simulink model "AngualarVelcoityToRepTests"  (Simulink 8.3)
settings: Solver=ode3  StartTime=0.0  StopTime=9.0  FixedStep=0.01  RelTol=1e-3
settings Model: Creator=user  LastModifiedBy=philip
settings OptimizationCC: ExpressionDepthLimit=2147483647
settings DebuggingCC: FcnCallInpInsideContextMsg=UseLocalSettings

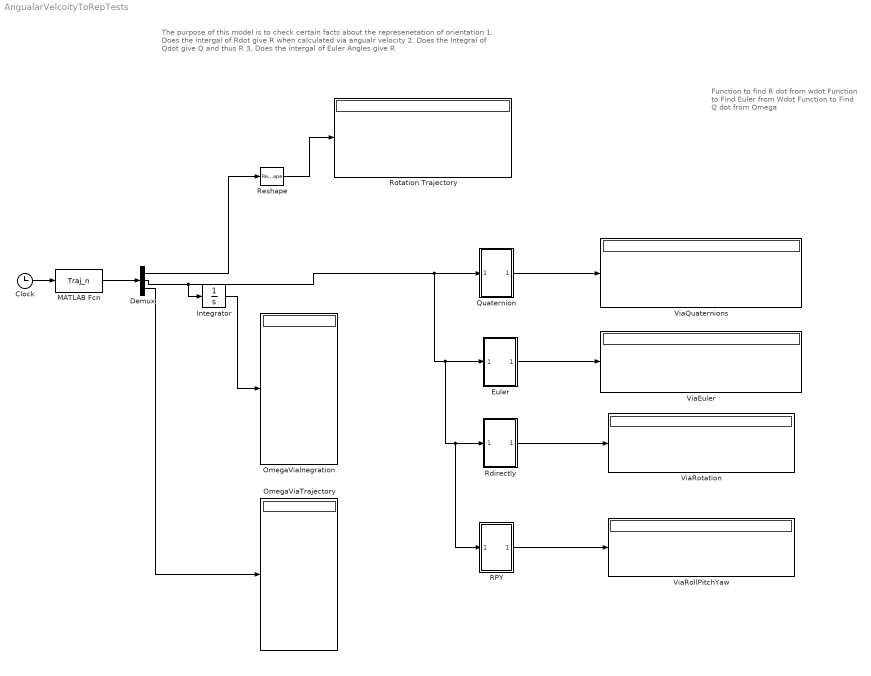
== system AngualarVelcoityToRepTests ==
  note: The purpose of this model is to check certain facts about the represenetation of orientation
      | 1. Does the intergal of Rdot give R when calculated via angualr velocity
      | 2.  Does the Integral of Qdot give Q and thus R
      | 3. Does the intergal of Euler Angles give R
  note: Function to find R dot from wdot
      | Function to Find Euler from Wdot
      | Function to Find Q dot from Omega
  Clock : Clock
  Demux : Demux  Outputs=[9 3 3]
  Euler : Subsystem
  Integrator : Integrator  InitialCondition=[0 0 0]
  MATLAB Fcn : MATLABFcn  MATLABFcn=Traj_n  OutputDimensions=15
  OmegaViaInegration : Display
  OmegaViaTrajectory : Display
  Quaternion : Subsystem
  RPY : Subsystem
  Rdirectly : Subsystem
  Reshape : Reshape  OutputDimensionality=Customize  OutputDimensions=[3,3]
  "Rotation Trajectory " : Display
  ViaEuler : Display
  ViaQuaternions : Display
  ViaRollPitchYaw : Display
  ViaRotation : Display
  wires:
  Clock/1 -> MATLAB Fcn/1
  Rdirectly/1(Out1) -> ViaRotation/1
  Euler/1(Out1) -> ViaEuler/1
  RPY/1(Out1) -> ViaRollPitchYaw/1
  MATLAB Fcn/1 -> Demux/1
  Integrator/1 -> OmegaViaInegration/1
  Quaternion/1(Out1) -> ViaQuaternions/1
  Demux/2 -> Integrator/1, RPY/1(In1), Rdirectly/1(In1), Euler/1(In1), Quaternion/1(In1)
  Demux/1 -> Reshape/1
  Demux/3 -> OmegaViaTrajectory/1
  Reshape/1 -> "Rotation Trajectory "/1

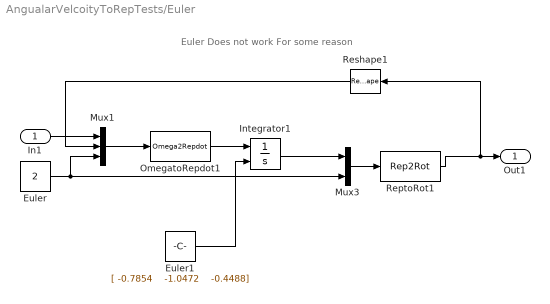
== system AngualarVelcoityToRepTests/Euler ==
  note: Euler Does not work For some reason
  In1 : Inport
  Euler : Constant  Value=2
  Euler1 : Constant  Value=|
      | [ -0.7854
      |    -1.0472
      |    -0.4488]
  Integrator1 : Integrator  InitialConditionSource=external
  Mux1 : Mux  Inputs=[3 9 1]
  Mux3 : Mux  Inputs=[3 1]
  OmegatoRepdot1 : MATLABFcn  MATLABFcn=Omega2Repdot  OutputDimensions=3
  ReptoRot1 : MATLABFcn  MATLABFcn=Rep2Rot  OutputDimensions=[3 3]  Output1D=off
  Reshape1 : Reshape
  Out1 : Outport
  wires:
  Mux1/1 -> OmegatoRepdot1/1
  Euler1/1 -> Integrator1/2
  OmegatoRepdot1/1 -> Integrator1/1
  ReptoRot1/1 -> Reshape1/1, Out1/1
  Reshape1/1 -> Mux1/2
  Euler/1 -> Mux1/3, Mux3/2
  Integrator1/1 -> Mux3/1
  Mux3/1 -> ReptoRot1/1
  In1/1 -> Mux1/1

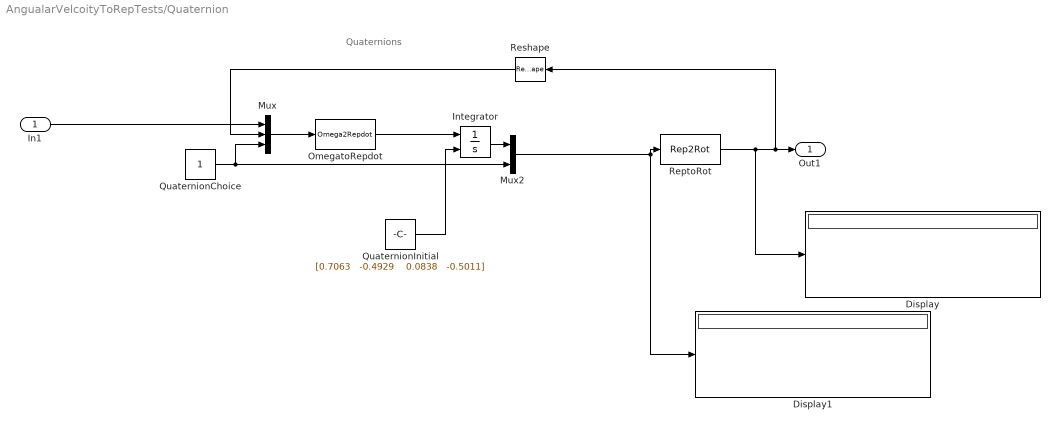
== system AngualarVelcoityToRepTests/Quaternion ==
  note: Quaternions
  In1 : Inport
  Display : Display
  Display1 : Display
  Integrator : Integrator  InitialConditionSource=external
  Mux : Mux  Inputs=[3 9 1]
  Mux2 : Mux  Inputs=[4 1]
  OmegatoRepdot : MATLABFcn  MATLABFcn=Omega2Repdot  OutputDimensions=4
  QuaternionChoice : Constant
  QuaternionInitial : Constant  Value="[0.7063   -0.4929    0.0838   -0.5011]"
  ReptoRot : MATLABFcn  MATLABFcn=Rep2Rot  OutputDimensions=[3 3]  Output1D=off
  Reshape : Reshape
  Out1 : Outport
  wires:
  Mux/1 -> OmegatoRepdot/1
  QuaternionInitial/1 -> Integrator/2
  OmegatoRepdot/1 -> Integrator/1
  ReptoRot/1 -> Display/1, Reshape/1, Out1/1
  Reshape/1 -> Mux/2
  QuaternionChoice/1 -> Mux/3, Mux2/2
  Integrator/1 -> Mux2/1
  Mux2/1 -> Display1/1, ReptoRot/1
  In1/1 -> Mux/1

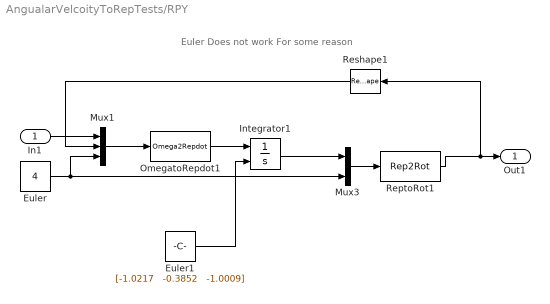
== system AngualarVelcoityToRepTests/RPY ==
  note: Euler Does not work For some reason
  In1 : Inport
  Euler : Constant  Value=4
  Euler1 : Constant  Value="[-1.0217   -0.3852   -1.0009]"
  Integrator1 : Integrator  InitialConditionSource=external
  Mux1 : Mux  Inputs=[3 9 1]
  Mux3 : Mux  Inputs=[3 1]
  OmegatoRepdot1 : MATLABFcn  MATLABFcn=Omega2Repdot  OutputDimensions=3
  ReptoRot1 : MATLABFcn  MATLABFcn=Rep2Rot  OutputDimensions=[3 3]  Output1D=off
  Reshape1 : Reshape
  Out1 : Outport
  wires:
  Mux1/1 -> OmegatoRepdot1/1
  Euler1/1 -> Integrator1/2
  OmegatoRepdot1/1 -> Integrator1/1
  ReptoRot1/1 -> Reshape1/1, Out1/1
  Reshape1/1 -> Mux1/2
  Euler/1 -> Mux1/3, Mux3/2
  Integrator1/1 -> Mux3/1
  Mux3/1 -> ReptoRot1/1
  In1/1 -> Mux1/1

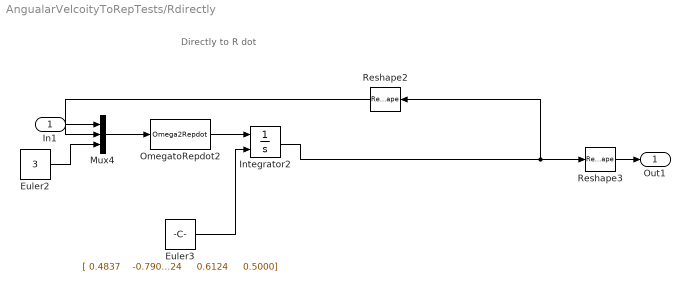
== system AngualarVelcoityToRepTests/Rdirectly ==
  note: Directly to R dot
  In1 : Inport
  Euler2 : Constant  Value=3
  Euler3 : Constant  Value=|
      | [ 0.4837
      |    -0.7905
      |     0.3758
      |     0.6253
      |     0.0117
      |    -0.7803
      |     0.6124
      |     0.6124
      |     0.5000]
  Integrator2 : Integrator  InitialConditionSource=external
  Mux4 : Mux  Inputs=[3 9 1]
  OmegatoRepdot2 : MATLABFcn  MATLABFcn=Omega2Repdot  OutputDimensions=9
  Reshape2 : Reshape
  Reshape3 : Reshape  OutputDimensionality=Customize  OutputDimensions=[3,3]
  Out1 : Outport
  wires:
  Mux4/1 -> OmegatoRepdot2/1
  Euler3/1 -> Integrator2/2
  OmegatoRepdot2/1 -> Integrator2/1
  Reshape2/1 -> Mux4/2
  Euler2/1 -> Mux4/3
  Integrator2/1 -> Reshape2/1, Reshape3/1
  In1/1 -> Mux4/1
  Reshape3/1 -> Out1/1
